simulink model "Model_Refrigeration_Constant"  (R2022a)
settings: Solver=VariableStepAuto  StartTime=0.0  StopTime=properties_8(15,2)  FixedStep=properties_8(14,2)  MaxStep=properties_8(14,2)  RelTol=1e-3  AbsTol=1e-3
InitFcn:
  | tube_D = 0.02; % [m] Refrigerant tube diameter
  | duct_W = 0.4; % [m] Air duct width
  | house_L = 4.5; % [m] House length
  | house_W = 3; % [m] House width
  | house_H = 2; % [m] House height
  | roof_pitch = 0; % [deg] Roof pitch
undefined symbols (not defined in the file or in its folder): alpha_h_ratio_NE, alpha_h_ratio_NW, alpha_h_ratio_SE, alpha_h_ratio_SW, area_furniture, area_roof, area_wall_exterior_NE, area_wall_exterior_NW, area_wall_exterior_SE, area_wall_exterior_SW, area_window, cp_furniture, cp_roof, cp_wall_exterior_NE, cp_wall_exterior_NW, cp_wall_exterior_SE, cp_wall_exterior_SW, cp_window, hc_furniture_interior, hc_roof_exterior, hc_roof_interior, hc_wall_exterior_NE, hc_wall_exterior_NW, hc_wall_exterior_SE, hc_wall_exterior_SW, hc_wall_interior_NE, hc_wall_interior_NW, hc_wall_interior_SE, hc_wall_interior_SW, hc_window_exterior, hc_window_interior, k_roof, k_wall_NE, k_wall_NW, k_wall_SE, k_wall_SW, k_window, l_roof, mass_furniture, pitch_roof, properties_8, Q_infiltration_latent, Q_infiltration_sensible, Q_latent_occupant_skin, Q_lights, Q_motor, Q_occupant, rho_roof, rho_wall_NE, rho_wall_NW, rho_wall_SE, rho_wall_SW, rho_window, SC, sigbuilder_block, T_env, T_house_init, T_init_furniture, T_set, thicnkess_roof ... (+11)
libraries: fl_lib x61, nesl_utility x15, simulink x1
(part 1 of 2)
CloseFcn:
  | try,close(h1_sscfluids_refrigeration),end
  | clear h1_sscfluids_refrigeration
  | try,close(h2_sscfluids_refrigeration),end
  | clear h2_sscfluids_refrigeration
  | try,close(h3_sscfluids_refrigeration),end
  | clear h3_sscfluids_refrigeration
  | Results
  | clear tout simlog_sscfluids_refrigeration
  | clear T_env RH_env T_house_init RH_house_init T_set
  | clear tube_D duct_W house_L house_W house_H roof_pitch
Description:
  | Refrigeration Cycle (Air Conditioning)
settings Model: Creator=The MathWorks, Inc.  LastModifiedBy=mluser
settings SolverCC: AutoScaleAbsTol=off  AlgebraicLoopSolver=TrustRegion  MaxZcPerStep=1
settings DataIOCC: ReturnWorkspaceOutputs=off
settings DebuggingCC: UnconnectedInputMsg=warning  UnconnectedOutputMsg=warning  UnconnectedLineMsg=warning  SymbolicDimsDataTypeCodeGenerationDiagnostic=none  SFMachineParentedDataDiag=warning
settings SFSimCC: CustomCodeUndefinedFunction=UseInterfaceOnly
settings RTWCC: DLArmComputeVersion=19.05
settings SimscapeCC: SimscapeLogType=all  SimscapeLogSimulationStatistics=on  SimscapeLogName=simlog_sscfluids_refrigeration  SimscapeLogDataHistory=10000

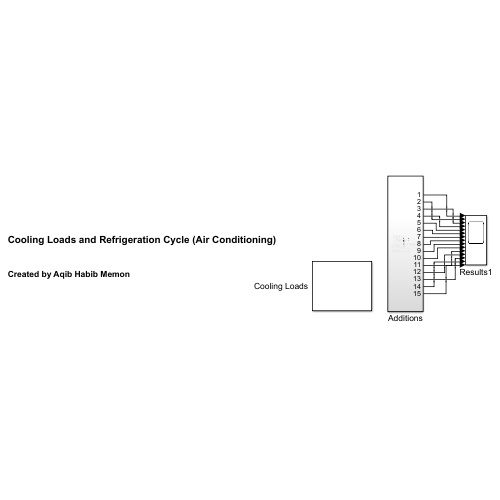
[thumbnail: Simulink's stored preview of the top-level diagram]
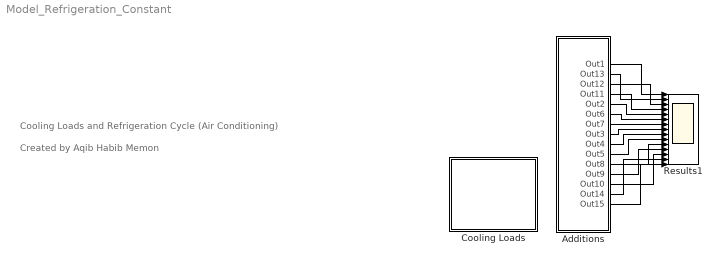
== system Model_Refrigeration_Constant ==
  note: Cooling Loads and Refrigeration Cycle (Air Conditioning)
  note: Created by Aqib Habib Memon
  Additions : Subsystem
  Cooling Loads : Subsystem
  Results1 : Scope  NumInputPorts=15
  wires:
  Additions/10(Out5) -> Results1/10
  Additions/9(Out4) -> Results1/9
  Additions/1(Out1) -> Results1/1
  Additions/2(Out13) -> Results1/2
  Additions/8(Out3) -> Results1/8
  Additions/7(Out7) -> Results1/7
  Additions/12(Out9) -> Results1/12
  Additions/5(Out2) -> Results1/5
  Additions/11(Out8) -> Results1/11
  Additions/6(Out6) -> Results1/6
  Additions/13(Out10) -> Results1/13
  Additions/3(Out12) -> Results1/3
  Additions/4(Out11) -> Results1/4
  Additions/14(Out14) -> Results1/14
  Additions/15(Out15) -> Results1/15

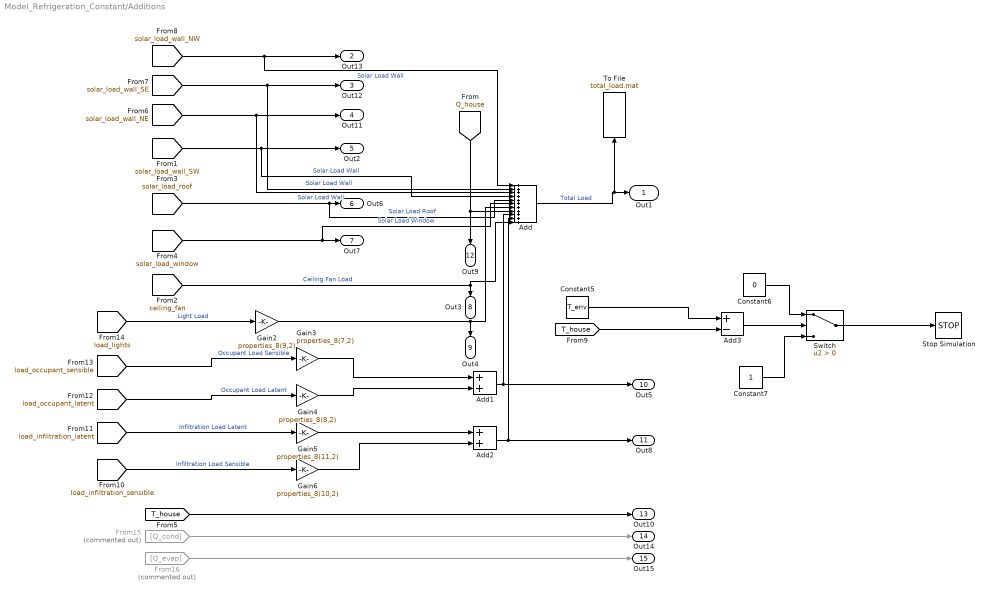
== system Model_Refrigeration_Constant/Additions ==
  Add : Sum  Inputs=+++++++++++
  Add1 : Sum
  Add2 : Sum
  Add3 : Sum  Inputs=+-
  Constant5 : Constant  Value=T_env
  Constant6 : Constant  Value=0
  Constant7 : Constant
  From15 : From  Commented=on  GotoTag=Q_cond
  From16 : From  Commented=on  GotoTag=Q_evap
  Gain2 : Gain  Gain=properties_8(9,2)
  Gain3 : Gain  Gain=properties_8(7,2)
  Gain4 : Gain  Gain=properties_8(8,2)
  Gain5 : Gain  Gain=properties_8(11,2)
  Gain6 : Gain  Gain=properties_8(10,2)
  Stop Simulation : Stop
  Switch : Switch  Criteria=u2 > Threshold  SaturateOnIntegerOverflow=off  InputSameDT=off
  To File : ToFile  Filename=total_load.mat  MatrixName=total_load
  Out1 : Outport
  Out13 : Outport  Port=2
  Out12 : Outport  Port=3
  Out11 : Outport  Port=4
  Out2 : Outport  Port=5
  Out6 : Outport  Port=6
  Out7 : Outport  Port=7
  Out3 : Outport  Port=8
  Out4 : Outport  Port=9
  Out5 : Outport  Port=10
  Out8 : Outport  Port=11
  Out9 : Outport  Port=12
  Out10 : Outport  Port=13
  Out14 : Outport  Port=14
  Out15 : Outport  Port=15
  wires:
  [load_lights] -> Gain2/1  "Light Load"
  [ceiling_fan] -> Add/11, Out3/1  "Ceiling Fan Load"
  Add/1 -> Out1/1, To File/1  "Total Load"
  [load_occupant_sensible] -> Gain3/1  "Occupant Load Sensible"
  [load_occupant_latent] -> Gain4/1  "Occupant Load Latent"
  [load_infiltration_sensible] -> Gain6/1  "Infiltration Load Sensible"
  [Q_house] -> Add/8, Out9/1
  [solar_load_wall_SW] -> Add/4, Out2/1  "Solar Load Wall"
  [solar_load_roof] -> Add/5, Out6/1  "Solar Load Roof"
  [solar_load_window] -> Add/6, Out7/1  "Solar Load Window"
  [T_house] -> Out10/1
  [solar_load_wall_NE] -> Add/3, Out11/1  "Solar Load Wall"
  [solar_load_wall_SE] -> Add/2, Out12/1  "Solar Load Wall"
  [solar_load_wall_NW] -> Add/1, Out13/1  "Solar Load Wall"
  [load_infiltration_latent] -> Gain5/1  "Infiltration Load Latent"
  Add1/1 -> Out5/1, Add/9
  Add2/1 -> Add/10, Out8/1
  Gain2/1 -> Add/7, Out4/1
  Gain3/1 -> Add1/1
  Gain4/1 -> Add1/2
  Gain5/1 -> Add2/1
  Gain6/1 -> Add2/2
  Constant5/1 -> Add3/1
  [T_house] -> Add3/2
  Add3/1 -> Switch/2
  Constant6/1 -> Switch/1
  Constant7/1 -> Switch/3
  Switch/1 -> Stop Simulation/1
  From16/1 -> Out15/1
  From15/1 -> Out14/1

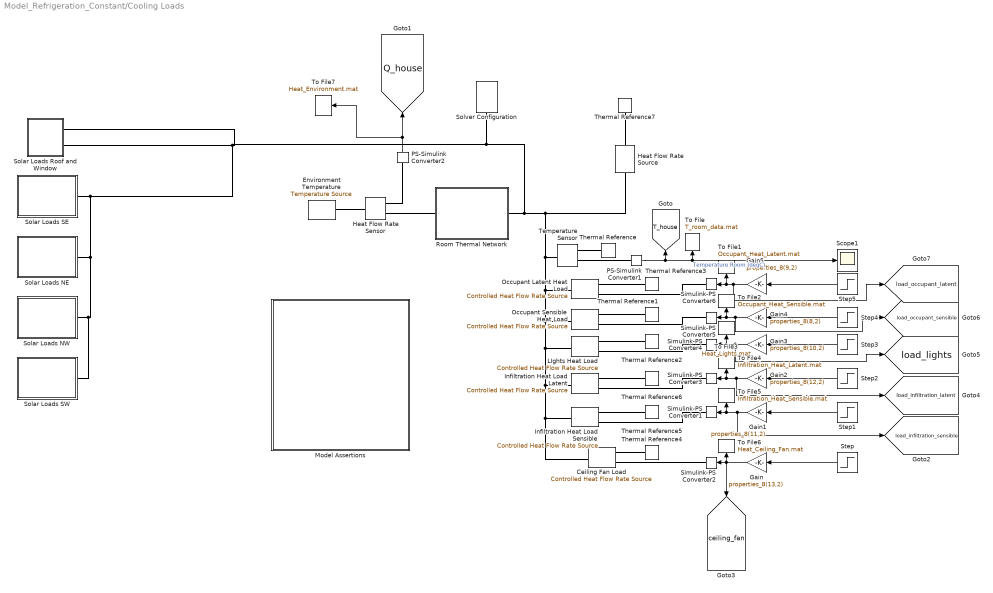
== system Model_Refrigeration_Constant/Cooling Loads ==
  Ceiling Fan Load : fl_lib/Thermal/Thermal Sources/Controlled Heat Flow Rate Source
      settings: SourceProductBaseCode=PW,SS,VE
  Environment Temperature : fl_lib/Thermal/Thermal Sources/Temperature Source  temperature=T_env degC
      settings: SourceProductBaseCode=PW,SS,VE
  Gain : Gain  Gain=properties_8(13,2)
  Gain1 : Gain  Gain=properties_8(11,2)
  Gain2 : Gain  Gain=properties_8(12,2)
  Gain3 : Gain  Gain=properties_8(10,2)
  Gain4 : Gain  Gain=properties_8(8,2)
  Gain5 : Gain  Gain=properties_8(9,2)
  Heat Flow Rate Sensor : fl_lib/Thermal/Thermal Sensors/Heat Flow Rate Sensor
      settings: SourceProductBaseCode=PW,SS,VE
  Heat Flow Rate Source : fl_lib/Thermal/Thermal Sources/Heat Flow Rate Source  heat_flow=5250 W
      settings: SourceProductBaseCode=PW,SS,VE  InternalSimscapePortConfiguration="{\"Bottom\":[],\"Left\":[{\"id\":\"B\",\"label\":\"B\",\"type\":\"foundation.thermal.thermal\"}],\"Right\":[{\"id\":\"A\",\"label\":\"A\",\"type\":\"foundation.thermal.thermal\"}],\"Top\":[]}"
  Infiltration Heat Load Latent : fl_lib/Thermal/Thermal Sources/Controlled Heat Flow Rate Source
      settings: SourceProductBaseCode=PW,SS,VE
  Infiltration Heat Load Sensible : fl_lib/Thermal/Thermal Sources/Controlled Heat Flow Rate Source
      settings: SourceProductBaseCode=PW,SS,VE
  LIghts Heat Load : fl_lib/Thermal/Thermal Sources/Controlled Heat Flow Rate Source
      settings: SourceProductBaseCode=PW,SS,VE
  Model Assertions : Subsystem
  Occupant Latent Heat Load : fl_lib/Thermal/Thermal Sources/Controlled Heat Flow Rate Source
      settings: SourceProductBaseCode=PW,SS,VE
  Occupant Sensible Heat Load : fl_lib/Thermal/Thermal Sources/Controlled Heat Flow Rate Source
      settings: SourceProductBaseCode=PW,SS,VE
  PS-Simulink Converter1 : nesl_utility/PS-Simulink Converter  PhysicalDomain=network_engine_domain  SubClassName=ps_output  LeftPortType=input  RightPortType=output  PseudoPeriodic=off  Frequencies=[]  VectorFormat=inherit  Unit=degC  AffineConversion=on
      settings: SourceProductBaseCode=SS,PW,VE
  PS-Simulink Converter2 : nesl_utility/PS-Simulink Converter  PhysicalDomain=network_engine_domain  SubClassName=ps_output  LeftPortType=input  RightPortType=output  PseudoPeriodic=off  Frequencies=[]  VectorFormat=inherit  Unit=W  AffineConversion=off
      settings: SourceProductBaseCode=SS,PW,VE
  Room Thermal Network : Subsystem  Tag=PublishSubsystem  mask(House Thermal Network){area_roof=l_roof * w_roof / (2*cosd(pitch_roof)), thickness_roof=thicnkess_roof, rho_roof=rho_roof, cp_roof=cp_roof, k_roof=k_roof, hc_roof_interior=hc_roof_interior, hc_roof_exterior=hc_roof_exterior, T_init_roof=T_house_init, area_wall_SE=area_wall_exterior_SE, thickness_wall_SE=thicnkess_wall_exterior_SE, rho_wall_SE=rho_wall_SE, cp_wall_SE=cp_wall_exterior_SE, k_wall_SE=k_wall_SE, hc_wall_interior_SE=hc_wall_interior_SE, hc_wall_exterior_SE=hc_wall_exterior_SE, T_init_wall_SE=T_house_init, area_wall_NE=area_wall_exterior_NE, thickness_wall_copy_NE=thicnkess_wall_exterior_NE, rho_wall_NE=rho_wall_NE, cp_wall_NE=cp_wall_exterior_NE, k_wall_NE=k_wall_NE, hc_wall_interior_NE=hc_wall_interior_NE, hc_wall_exterior_NE=hc_wall_exterior_NE, T_init_wall_NE=T_house_init, area_wall_SW=area_wall_exterior_SW, thickness_wall_SW=thicnkess_wall_exterior_SW, rho_wal_SW=rho_wall_SW, cp_wall_SW=cp_wall_exterior_SW, k_wall_SW=k_wall_SW, hc_wall_SW=hc_wall_interior_SW, hc_wall_exterior_SW=hc_wall_exterior_SW, T_init_wall_SW=T_house_init, area_wall_NW=area_wall_exterior_NW, thickness_wall_NW=thicnkess_wall_exterior_NW, rho_wall_NW=rho_wall_NW, cp_wall_NW=cp_wall_exterior_NW, k_wall_NW=k_wall_NW, hc_wall_interior_NW=hc_wall_interior_NW, hc_wall_exterior_NW=hc_wall_exterior_NW, T_init_wall_NW=T_house_init, area_window=area_window, thickness_window=thicnkess_window, rho_window=rho_window, cp_window=cp_window, k_window=k_window, hc_window_interior=hc_window_interior, hc_window_exterior=hc_window_exterior, T_init_window=T_house_init, area_furniture=area_furniture, M_furniture=mass_furniture, cp_furniture=cp_furniture, hc_furniture_interior=hc_furniture_interior, T_init_furniture=T_init_furniture}
      mask prompts: area_roof "Total area (m^2)"; thickness_roof "Average thickness (m)"; rho_roof "Average density (kg/m^3)"; cp_roof "Average specific heat (J/kg/K)"; k_roof "Average conductivity (W/m/K)"; hc_roof_interior "Interior heat transfer coefficient (W/m^2/K)"; hc_roof_exterior "Exterior heat transfer coefficient (W/m^2/K)"; T_init_roof "Initial temperature (degC)"; area_wall_SE "Total area (m^2)"; thickness_wall_SE "Average thickness (m)"; rho_wall_SE "Average density (kg/m^3)"; cp_wall_SE "Average specific heat (J/kg/K)"; k_wall_SE "Average conductivity (W/m/K)"; hc_wall_interior_SE "Interior heat transfer coefficient (W/m^2/K)"; hc_wall_exterior_SE "Exterior heat transfer coefficient (W/m^2/K)"; T_init_wall_SE "Initial temperature (degC)"; area_wall_NE "Total area (m^2)"; thickness_wall_copy_NE "Average thickness (m)"; rho_wall_NE "Average density (kg/m^3)"; cp_wall_NE "Average specific heat (J/kg/K)"; k_wall_NE "Average conductivity (W/m/K)"; hc_wall_interior_NE "Interior heat transfer coefficient (W/m^2/K)"; hc_wall_exterior_NE "Exterior heat transfer coefficient (W/m^2/K)"; T_init_wall_NE "Initial temperature (degC)"; area_wall_SW "Total area (m^2)"; thickness_wall_SW "Average thickness (m)"; rho_wal_SW "Average density (kg/m^3)"; cp_wall_SW "Average specific heat (J/kg/K)"; k_wall_SW "Average conductivity (W/m/K)"; hc_wall_SW "Interior heat transfer coefficient (W/m^2/K)"; hc_wall_exterior_SW "Exterior heat transfer coefficient (W/m^2/K)"; T_init_wall_SW "Initial temperature (degC)"; area_wall_NW "Total area (m^2)"; thickness_wall_NW "Average thickness (m)"; rho_wall_NW "Average density (kg/m^3)"; cp_wall_NW "Average specific heat (J/kg/K)"; k_wall_NW "Average conductivity (W/m/K)"; hc_wall_interior_NW "Interior heat transfer coefficient (W/m^2/K)"; hc_wall_exterior_NW "Exterior heat transfer coefficient (W/m^2/K)"; T_init_wall_NW "Initial temperature (degC)"; area_window "Total area (m^2)"; thickness_window "Average thickness (m)"; rho_window "Average density (kg/m^3)"; cp_window "Average specific heat (J/kg/K)"; k_window "Average conductivity (W/m/K)"; hc_window_interior "Interior heat transfer coefficient (W/m^2/K)"; hc_window_exterior "Exterior heat transfer coefficient (W/m^2/K)"; T_init_window "Initial temperature (degC)"; area_furniture "Total surface area (m^2)"; M_furniture "Total mass (kg)"; cp_furniture "Average specific heat (J/kg/K)"; hc_furniture_interior "Interior heat transfer coefficient (W/m^2/K)"; T_init_furniture "Initial temperature (degC)"
      mask help: This subsystem models heat transfer between the air in the interior of the house and the external environment.
      mask DialogControl TabRoof Prompt: Roof
      mask DialogControl TabWallSE Prompt: South East Walls
      mask DialogControl TabWallNE Prompt: North East Walls
      mask DialogControl TabWallSW Prompt: South West Walls
      mask DialogControl TabWallNW Prompt: North West Walls
      mask DialogControl TabWindow Prompt: Windows
      mask DialogControl TabFurniture Prompt: Furniture
  Scope1 : Scope
  Simulink-PS Converter{1..6} (6 alike) : nesl_utility/Simulink-PS Converter  PhysicalDomain=network_engine_domain  SubClassName=ps_input  LeftPortType=input  RightPortType=output  PseudoPeriodic=off  Frequencies=[]  NoiseDistribution=none  NoiseParameters=[]  Unit=1  AffineConversion=off  FilteringAndDerivatives=provide  SimscapeFilterOrder=1  InputFilterTimeConstant=0.001  UdotUserProvided=0
      settings: SourceProductBaseCode=SS,PW,VE
  Solar Loads NE : Subsystem
  Solar Loads NW : Subsystem
  Solar Loads Roof and Window : Subsystem
  Solar Loads SE : Subsystem
  Solar Loads SW : Subsystem
  Solver Configuration : nesl_utility/Solver Configuration  PhysicalDomain=network_engine_domain  SubClassName=solver  LeftPortType=input  RightPortType=generic  Tones=[]  Harmonics=[]  SimulateNoise=off  Profile=off  UseLocalSampling=off  EnableSwitchedLinearOptims=on  FrequencyDomain=off  UseCCode=off  RelTol=0.001  AbsTol=0.001  MinStep=1e-09  ToWorkspace=off  RevertToSquareIcSolve=off  NumHomotopyIterations=100  PhasorMode=off  PhasorModeNumHarmonics=1  IndexReductionMethod=DerivativeReplacement  DoDC=off  ResidualTolerance=1e-09  UseLocalSolver=off  LocalSolverChoice=NE_BACKWARD_EULER_ADVANCER  LocalSolverSampleTime=0.001  DoFixedCost=off  MaxNonlinIter=3  MaxModeIter=2  ComputeImpulses=off  ImpulseIterations=2  LinearAlgebra=auto  LinearAlgebraNumThread=0  EquationFormulation=NE_TIME_EF  DelaysMemoryBudget=1024  AutomaticFiltering=on  FilteringTimeConstant=0.001  PartitionStorageMethod=AS_NEEDED  PartitionMemoryBudget=1024  PartitionMethod=ROBUST
      settings: SourceProductBaseCode=SS,PW,VE
  Step : Step  Time=0  After=Q_motor  SampleTime=0
  Step1 : Step  Time=0  After=Q_infiltration_sensible  SampleTime=0
  Step2 : Step  Time=0  After=Q_infiltration_latent  SampleTime=0
  Step3 : Step  Time=0  After=Q_lights  SampleTime=0
  Step4 : Step  Time=0  After=Q_occupant  SampleTime=0
  Step5 : Step  Time=0  After=Q_latent_occupant_skin  SampleTime=0
  Temperature Sensor : fl_lib/Thermal/Thermal Sensors/Temperature Sensor
      settings: SourceProductBaseCode=PW,SS,VE
  Thermal Reference{,1..7} (8 alike) : fl_lib/Thermal/Thermal Elements/Thermal Reference
      settings: SourceProductBaseCode=PW,SS,VE
  To File : ToFile  Filename=T_room_data.mat  MatrixName=T_room_data
  To File1 : ToFile  Filename=Occupant_Heat_Latent.mat  MatrixName=Occupant_Heat_Latent
  To File2 : ToFile  Filename=Occupant_Heat_Sensible.mat  MatrixName=Occupant_Heat_Sensible
  To File3 : ToFile  Filename=Heat_Lights.mat  MatrixName=Heat_Lights
  To File4 : ToFile  Filename=Infiltration_Heat_Latent.mat  MatrixName=Infiltration_Heat_Latent
  To File5 : ToFile  Filename=Infiltration_Heat_Sensible.mat  MatrixName=Infiltration_Heat_Sensible
  To File6 : ToFile  Filename=Heat_Ceiling_Fan.mat  MatrixName=Heat_Ceiling_Fan
  To File7 : ToFile  Filename=Heat_Environment.mat  MatrixName=Heat_Environment
  tag scope: Q_house=global, T_house=global, ceiling_fan=global, load_infiltration_latent=global, load_infiltration_sensible=global, load_lights=global, load_occupant_latent=global, load_occupant_sensible=global
  wires:
  PS-Simulink Converter1/1 -> Scope1/1, To File/1, [T_house]  "Temperature Room (degC)"
  PS-Simulink Converter2/1 -> To File7/1, [Q_house]
  Gain/1 -> To File6/1, [ceiling_fan], Simulink-PS Converter2/1
  Step/1 -> Gain/1
  Step1/1 -> Gain1/1
  Step2/1 -> Gain2/1
  Step3/1 -> Gain3/1
  Step4/1 -> Gain4/1
  Step5/1 -> Gain5/1
  Gain5/1 -> Simulink-PS Converter6/1, To File1/1, [load_occupant_latent]
  Gain4/1 -> [load_occupant_sensible], To File2/1, Simulink-PS Converter5/1
  Gain3/1 -> [load_lights], To File3/1, Simulink-PS Converter4/1
  Gain2/1 -> [load_infiltration_latent], To File4/1, Simulink-PS Converter3/1
  Gain1/1 -> [load_infiltration_sensible], To File5/1, Simulink-PS Converter1/1
  connections:
  Temperature Sensor/RConn2 -- PS-Simulink Converter1/LConn1
  Temperature Sensor/RConn1 -- Thermal Reference/LConn1
  Solar Loads SW/RConn1 -- Solar Loads NW/RConn1 -- Solar Loads NE/RConn1 -- Solar Loads Roof and Window/RConn1 -- Solver Configuration/RConn1 -- Heat Flow Rate Source/RConn1 -- Ceiling Fan Load/LConn1 -- Infiltration Heat Load Sensible/LConn1 -- Infiltration Heat Load Latent/LConn1 -- LIghts Heat Load/LConn1 -- Occupant Sensible Heat Load/LConn1 -- Occupant Latent Heat Load/LConn1 -- Temperature Sensor/LConn1 -- Room Thermal Network/RConn1 -- Solar Loads Roof and Window/RConn2 -- Solar Loads SE/RConn1
  Thermal Reference4/LConn1 -- Ceiling Fan Load/RConn2
  Simulink-PS Converter2/RConn1 -- Ceiling Fan Load/RConn1
  Heat Flow Rate Sensor/LConn1 -- Environment Temperature/LConn1
  PS-Simulink Converter2/LConn1 -- Heat Flow Rate Sensor/RConn1
  Occupant Latent Heat Load/RConn2 -- Thermal Reference3/LConn1
  Occupant Sensible Heat Load/RConn2 -- Thermal Reference1/LConn1
  LIghts Heat Load/RConn2 -- Thermal Reference2/LConn1
  Infiltration Heat Load Sensible/RConn2 -- Thermal Reference5/LConn1
  Thermal Reference6/LConn1 -- Infiltration Heat Load Latent/RConn2
  Simulink-PS Converter6/RConn1 -- Occupant Latent Heat Load/RConn1
  Simulink-PS Converter5/RConn1 -- Occupant Sensible Heat Load/RConn1
  Simulink-PS Converter4/RConn1 -- LIghts Heat Load/RConn1
  Simulink-PS Converter3/RConn1 -- Infiltration Heat Load Latent/RConn1
  Simulink-PS Converter1/RConn1 -- Infiltration Heat Load Sensible/RConn1
  Heat Flow Rate Sensor/RConn2 -- Room Thermal Network/LConn1
  Thermal Reference7/LConn1 -- Heat Flow Rate Source/LConn1

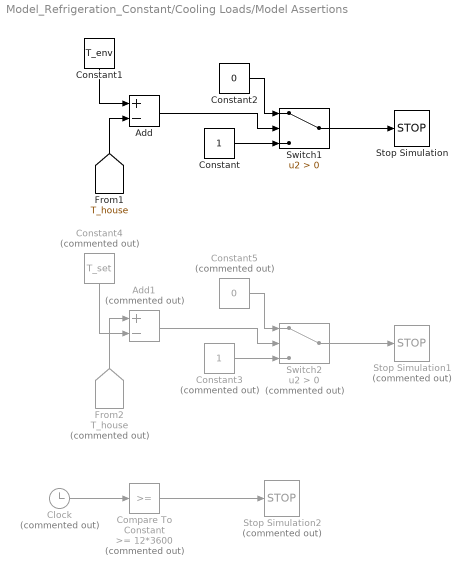
== system Model_Refrigeration_Constant/Cooling Loads/Model Assertions ==
  Add : Sum  Inputs=+-
  Add1 : Sum  Commented=on  Inputs=+-
  Clock : Clock  Commented=on
  Compare To Constant : simulink/Logic and Bit Operations/Compare To Constant  Commented=on  relop=>=  const=12*3600  OutDataTypeStr=boolean
  Constant : Constant
  Constant1 : Constant  Value=T_env
  Constant2 : Constant  Value=0
  Constant3 : Constant  Commented=on
  Constant4 : Constant  Commented=on  Value=T_set
  Constant5 : Constant  Commented=on  Value=0
  From2 : From  Commented=on  GotoTag=T_house  TagVisibility=global
  Stop Simulation : Stop
  Stop Simulation1 : Stop  Commented=on
  Stop Simulation2 : Stop  Commented=on
  Switch1 : Switch  Criteria=u2 > Threshold  SaturateOnIntegerOverflow=off  InputSameDT=off
  Switch2 : Switch  Commented=on  Criteria=u2 > Threshold  SaturateOnIntegerOverflow=off  InputSameDT=off
  wires:
  Constant/1 -> Switch1/3
  Constant3/1 -> Switch2/3
  [T_house] -> Add/2
  Constant4/1 -> Add1/2
  Constant2/1 -> Switch1/1
  Switch1/1 -> Stop Simulation/1
  Add1/1 -> Switch2/2
  Constant5/1 -> Switch2/1
  Add/1 -> Switch1/2
  Switch2/1 -> Stop Simulation1/1
  Constant1/1 -> Add/1
  From2/1 -> Add1/1
  Compare To Constant/1 -> Stop Simulation2/1
  Clock/1 -> Compare To Constant/1

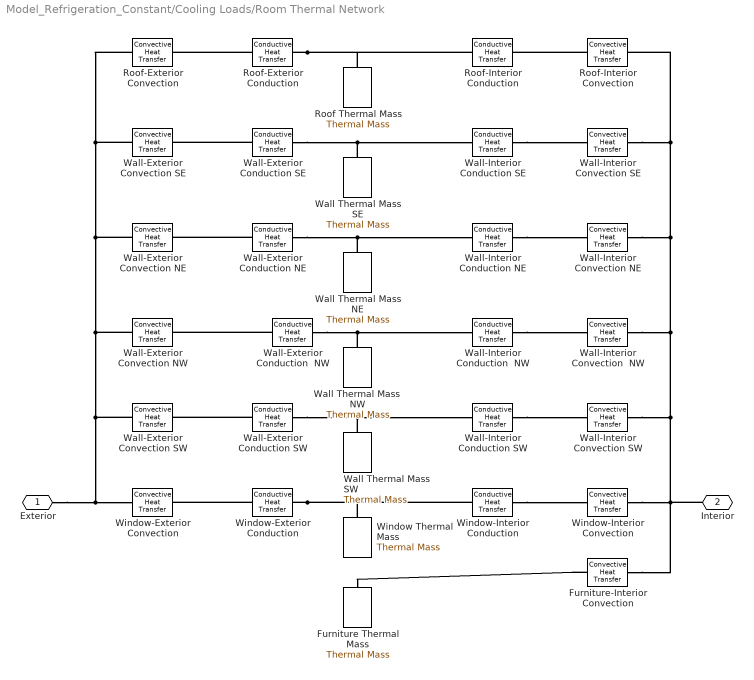
== system Model_Refrigeration_Constant/Cooling Loads/Room Thermal Network ==
  Furniture Thermal Mass : fl_lib/Thermal/Thermal Elements/Thermal Mass  mass=M_furniture kg  sp_heat=cp_furniture J/(K*kg)  T_specify=on  T_priority=High  T=T_init_furniture degC  T_nominal_specify=off  T_nominal_unit=K  T_nominal_value=1  Q_specify=off  Q_priority=None  Q=0 W  Q_nominal_specify=off  Q_nominal_unit=W  Q_nominal_value=1
      settings: SourceProductBaseCode=PW,SS,VE
  Furniture-Interior Convection : fl_lib/Thermal/Thermal Elements/Convective Heat Transfer  area=area_furniture m^2  heat_tr_coeff=hc_furniture_interior W/(K*m^2)  T_specify=off  T_priority=None  T=0 K  T_nominal_specify=off  T_nominal_unit=K  T_nominal_value=1  Q_specify=off  Q_priority=None  Q=0 W  Q_nominal_specify=off  Q_nominal_unit=W  Q_nominal_value=1
      settings: SourceProductBaseCode=PW,SS,VE
  Roof Thermal Mass : fl_lib/Thermal/Thermal Elements/Thermal Mass  mass=rho_roof * area_roof * thickness_roof kg  sp_heat=cp_roof J/(K*kg)  T_specify=on  T_priority=High  T=T_init_roof degC  T_nominal_specify=off  T_nominal_unit=K  T_nominal_value=1  Q_specify=off  Q_priority=None  Q=0 W  Q_nominal_specify=off  Q_nominal_unit=W  Q_nominal_value=1
      settings: SourceProductBaseCode=PW,SS,VE
  Roof-Exterior Conduction : fl_lib/Thermal/Thermal Elements/Conductive Heat Transfer  area=area_roof m^2  thickness=thickness_roof / 2 m  th_cond=k_roof W/(K*m)  T_specify=off  T_priority=None  T=0 K  T_nominal_specify=off  T_nominal_unit=K  T_nominal_value=1  Q_specify=off  Q_priority=None  Q=0 W  Q_nominal_specify=off  Q_nominal_unit=W  Q_nominal_value=1
      settings: SourceProductBaseCode=PW,SS,VE
  Roof-Exterior Convection : fl_lib/Thermal/Thermal Elements/Convective Heat Transfer  area=area_roof m^2  heat_tr_coeff=hc_roof_exterior W/(K*m^2)  T_specify=off  T_priority=None  T=0 K  T_nominal_specify=off  T_nominal_unit=K  T_nominal_value=1  Q_specify=off  Q_priority=None  Q=0 W  Q_nominal_specify=off  Q_nominal_unit=W  Q_nominal_value=1
      settings: SourceProductBaseCode=PW,SS,VE
  Roof-Interior Conduction : fl_lib/Thermal/Thermal Elements/Conductive Heat Transfer  area=area_roof m^2  thickness=thickness_roof / 2 m  th_cond=k_roof W/(K*m)  T_specify=off  T_priority=None  T=0 K  T_nominal_specify=off  T_nominal_unit=K  T_nominal_value=1  Q_specify=off  Q_priority=None  Q=0 W  Q_nominal_specify=off  Q_nominal_unit=W  Q_nominal_value=1
      settings: SourceProductBaseCode=PW,SS,VE
  Roof-Interior Convection : fl_lib/Thermal/Thermal Elements/Convective Heat Transfer  area=area_roof m^2  heat_tr_coeff=hc_roof_interior W/(K*m^2)  T_specify=off  T_priority=None  T=0 K  T_nominal_specify=off  T_nominal_unit=K  T_nominal_value=1  Q_specify=off  Q_priority=None  Q=0 W  Q_nominal_specify=off  Q_nominal_unit=W  Q_nominal_value=1
      settings: SourceProductBaseCode=PW,SS,VE
  Wall Thermal Mass  NW : fl_lib/Thermal/Thermal Elements/Thermal Mass  mass=mass_wall_exterior_NW kg  sp_heat=cp_wall_NW J/(K*kg)  T_specify=on  T_priority=High  T=T_init_wall_NW degC  T_nominal_specify=off  T_nominal_unit=K  T_nominal_value=1  Q_specify=off  Q_priority=None  Q=0 W  Q_nominal_specify=off  Q_nominal_unit=W  Q_nominal_value=1
      settings: SourceProductBaseCode=PW,SS,VE
  Wall Thermal Mass NE : fl_lib/Thermal/Thermal Elements/Thermal Mass  mass=mass_wall_exterior_NE kg  sp_heat=cp_wall_NE J/(K*kg)  T_specify=on  T_priority=High  T=T_init_wall_NE degC  T_nominal_specify=off  T_nominal_unit=K  T_nominal_value=1  Q_specify=off  Q_priority=None  Q=0 W  Q_nominal_specify=off  Q_nominal_unit=W  Q_nominal_value=1
      settings: SourceProductBaseCode=PW,SS,VE
  Wall Thermal Mass SE : fl_lib/Thermal/Thermal Elements/Thermal Mass  mass=mass_wall_exterior_SE kg  sp_heat=cp_wall_SE J/(K*kg)  T_specify=on  T_priority=High  T=T_init_wall_SE degC  T_nominal_specify=off  T_nominal_unit=K  T_nominal_value=1  Q_specify=off  Q_priority=None  Q=0 W  Q_nominal_specify=off  Q_nominal_unit=W  Q_nominal_value=1
      settings: SourceProductBaseCode=PW,SS,VE
  Wall Thermal Mass SW : fl_lib/Thermal/Thermal Elements/Thermal Mass  mass=mass_wall_exterior_SW kg  sp_heat=cp_wall_SW J/(K*kg)  T_specify=on  T_priority=High  T=T_init_wall_SW degC  T_nominal_specify=off  T_nominal_unit=K  T_nominal_value=1  Q_specify=off  Q_priority=None  Q=0 W  Q_nominal_specify=off  Q_nominal_unit=W  Q_nominal_value=1
      settings: SourceProductBaseCode=PW,SS,VE
  Wall-Exterior Conduction  NW : fl_lib/Thermal/Thermal Elements/Conductive Heat Transfer  area=area_wall_NW m^2  thickness=thicnkess_wall_exterior_NW / 2 m  th_cond=k_wall_NW W/(K*m)  T_specify=off  T_priority=None  T=0 K  T_nominal_specify=off  T_nominal_unit=K  T_nominal_value=1  Q_specify=off  Q_priority=None  Q=0 W  Q_nominal_specify=off  Q_nominal_unit=W  Q_nominal_value=1
      settings: SourceProductBaseCode=PW,SS,VE
  Wall-Exterior Conduction NE : fl_lib/Thermal/Thermal Elements/Conductive Heat Transfer  area=area_wall_NE m^2  thickness=thicnkess_wall_exterior_NE / 2 m  th_cond=k_wall_NE W/(K*m)  T_specify=off  T_priority=None  T=0 K  T_nominal_specify=off  T_nominal_unit=K  T_nominal_value=1  Q_specify=off  Q_priority=None  Q=0 W  Q_nominal_specify=off  Q_nominal_unit=W  Q_nominal_value=1
      settings: SourceProductBaseCode=PW,SS,VE
  Wall-Exterior Conduction SE : fl_lib/Thermal/Thermal Elements/Conductive Heat Transfer  area=area_wall_SE m^2  thickness=thicnkess_wall_exterior_SE / 2 m  th_cond=k_wall_SE W/(K*m)  T_specify=off  T_priority=None  T=0 K  T_nominal_specify=off  T_nominal_unit=K  T_nominal_value=1  Q_specify=off  Q_priority=None  Q=0 W  Q_nominal_specify=off  Q_nominal_unit=W  Q_nominal_value=1
      settings: SourceProductBaseCode=PW,SS,VE
  Wall-Exterior Conduction SW : fl_lib/Thermal/Thermal Elements/Conductive Heat Transfer  area=area_wall_SW m^2  thickness=thicnkess_wall_exterior_SW / 2 m  th_cond=k_wall_SW W/(K*m)  T_specify=off  T_priority=None  T=0 K  T_nominal_specify=off  T_nominal_unit=K  T_nominal_value=1  Q_specify=off  Q_priority=None  Q=0 W  Q_nominal_specify=off  Q_nominal_unit=W  Q_nominal_value=1
      settings: SourceProductBaseCode=PW,SS,VE
  Wall-Exterior Convection NE : fl_lib/Thermal/Thermal Elements/Convective Heat Transfer  area=area_wall_NE m^2  heat_tr_coeff=hc_wall_exterior_NE W/(K*m^2)  T_specify=off  T_priority=None  T=0 K  T_nominal_specify=off  T_nominal_unit=K  T_nominal_value=1  Q_specify=off  Q_priority=None  Q=0 W  Q_nominal_specify=off  Q_nominal_unit=W  Q_nominal_value=1
      settings: SourceProductBaseCode=PW,SS,VE
  Wall-Exterior Convection NW : fl_lib/Thermal/Thermal Elements/Convective Heat Transfer  area=area_wall_NW m^2  heat_tr_coeff=hc_wall_exterior_NW W/(K*m^2)  T_specify=off  T_priority=None  T=0 K  T_nominal_specify=off  T_nominal_unit=K  T_nominal_value=1  Q_specify=off  Q_priority=None  Q=0 W  Q_nominal_specify=off  Q_nominal_unit=W  Q_nominal_value=1
      settings: SourceProductBaseCode=PW,SS,VE
  Wall-Exterior Convection SE : fl_lib/Thermal/Thermal Elements/Convective Heat Transfer  area=area_wall_SE m^2  heat_tr_coeff=hc_wall_exterior_SE W/(K*m^2)  T_specify=off  T_priority=None  T=0 K  T_nominal_specify=off  T_nominal_unit=K  T_nominal_value=1  Q_specify=off  Q_priority=None  Q=0 W  Q_nominal_specify=off  Q_nominal_unit=W  Q_nominal_value=1
      settings: SourceProductBaseCode=PW,SS,VE
  Wall-Exterior Convection SW : fl_lib/Thermal/Thermal Elements/Convective Heat Transfer  area=area_wall_SW m^2  heat_tr_coeff=hc_wall_exterior_SW W/(K*m^2)  T_specify=off  T_priority=None  T=0 K  T_nominal_specify=off  T_nominal_unit=K  T_nominal_value=1  Q_specify=off  Q_priority=None  Q=0 W  Q_nominal_specify=off  Q_nominal_unit=W  Q_nominal_value=1
      settings: SourceProductBaseCode=PW,SS,VE
  Wall-Interior Conduction  NW : fl_lib/Thermal/Thermal Elements/Conductive Heat Transfer  area=area_wall_NW m^2  thickness=thicnkess_wall_exterior_NW/ 2 m  th_cond=k_wall_NW W/(K*m)  T_specify=off  T_priority=None  T=0 K  T_nominal_specify=off  T_nominal_unit=K  T_nominal_value=1  Q_specify=off  Q_priority=None  Q=0 W  Q_nominal_specify=off  Q_nominal_unit=W  Q_nominal_value=1
      settings: SourceProductBaseCode=PW,SS,VE
  Wall-Interior Conduction NE : fl_lib/Thermal/Thermal Elements/Conductive Heat Transfer  area=area_wall_NE m^2  thickness=thicnkess_wall_exterior_NE/ 2 m  th_cond=k_wall_NE W/(K*m)  T_specify=off  T_priority=None  T=0 K  T_nominal_specify=off  T_nominal_unit=K  T_nominal_value=1  Q_specify=off  Q_priority=None  Q=0 W  Q_nominal_specify=off  Q_nominal_unit=W  Q_nominal_value=1
      settings: SourceProductBaseCode=PW,SS,VE
  Wall-Interior Conduction SE : fl_lib/Thermal/Thermal Elements/Conductive Heat Transfer  area=area_wall_SE m^2  thickness=thicnkess_wall_exterior_SE/ 2 m  th_cond=k_wall_SE W/(K*m)  T_specify=off  T_priority=None  T=0 K  T_nominal_specify=off  T_nominal_unit=K  T_nominal_value=1  Q_specify=off  Q_priority=None  Q=0 W  Q_nominal_specify=off  Q_nominal_unit=W  Q_nominal_value=1
      settings: SourceProductBaseCode=PW,SS,VE
  Wall-Interior Conduction SW : fl_lib/Thermal/Thermal Elements/Conductive Heat Transfer  area=area_wall_SW m^2  thickness=thicnkess_wall_exterior_SW/ 2 m  th_cond=k_wall_SW W/(K*m)  T_specify=off  T_priority=None  T=0 K  T_nominal_specify=off  T_nominal_unit=K  T_nominal_value=1  Q_specify=off  Q_priority=None  Q=0 W  Q_nominal_specify=off  Q_nominal_unit=W  Q_nominal_value=1
      settings: SourceProductBaseCode=PW,SS,VE
  Wall-Interior Convection  NW : fl_lib/Thermal/Thermal Elements/Convective Heat Transfer  area=area_wall_NW m^2  heat_tr_coeff=hc_wall_interior_NW W/(K*m^2)  T_specify=off  T_priority=None  T=0 K  T_nominal_specify=off  T_nominal_unit=K  T_nominal_value=1  Q_specify=off  Q_priority=None  Q=0 W  Q_nominal_specify=off  Q_nominal_unit=W  Q_nominal_value=1
      settings: SourceProductBaseCode=PW,SS,VE
  Wall-Interior Convection NE : fl_lib/Thermal/Thermal Elements/Convective Heat Transfer  area=area_wall_NE m^2  heat_tr_coeff=hc_wall_interior_NE W/(K*m^2)  T_specify=off  T_priority=None  T=0 K  T_nominal_specify=off  T_nominal_unit=K  T_nominal_value=1  Q_specify=off  Q_priority=None  Q=0 W  Q_nominal_specify=off  Q_nominal_unit=W  Q_nominal_value=1
      settings: SourceProductBaseCode=PW,SS,VE
  Wall-Interior Convection SE : fl_lib/Thermal/Thermal Elements/Convective Heat Transfer  area=area_wall_SE m^2  heat_tr_coeff=hc_wall_interior_SE W/(K*m^2)  T_specify=off  T_priority=None  T=0 K  T_nominal_specify=off  T_nominal_unit=K  T_nominal_value=1  Q_specify=off  Q_priority=None  Q=0 W  Q_nominal_specify=off  Q_nominal_unit=W  Q_nominal_value=1
      settings: SourceProductBaseCode=PW,SS,VE
  Wall-Interior Convection SW : fl_lib/Thermal/Thermal Elements/Convective Heat Transfer  area=area_wall_SW m^2  heat_tr_coeff=hc_wall_interior_SW W/(K*m^2)  T_specify=off  T_priority=None  T=0 K  T_nominal_specify=off  T_nominal_unit=K  T_nominal_value=1  Q_specify=off  Q_priority=None  Q=0 W  Q_nominal_specify=off  Q_nominal_unit=W  Q_nominal_value=1
      settings: SourceProductBaseCode=PW,SS,VE
  Window Thermal Mass : fl_lib/Thermal/Thermal Elements/Thermal Mass  mass=rho_window * area_window * thickness_window kg  sp_heat=cp_window J/(K*kg)  T_specify=on  T_priority=High  T=T_init_window degC  T_nominal_specify=off  T_nominal_unit=K  T_nominal_value=1  Q_specify=off  Q_priority=None  Q=0 W  Q_nominal_specify=off  Q_nominal_unit=W  Q_nominal_value=1
      settings: SourceProductBaseCode=PW,SS,VE
  Window-Exterior Conduction : fl_lib/Thermal/Thermal Elements/Conductive Heat Transfer  area=area_window m^2  thickness=thickness_window / 2 m  th_cond=k_window W/(K*m)  T_specify=off  T_priority=None  T=0 K  T_nominal_specify=off  T_nominal_unit=K  T_nominal_value=1  Q_specify=off  Q_priority=None  Q=0 W  Q_nominal_specify=off  Q_nominal_unit=W  Q_nominal_value=1
      settings: SourceProductBaseCode=PW,SS,VE
  Window-Exterior Convection : fl_lib/Thermal/Thermal Elements/Convective Heat Transfer  area=area_window m^2  heat_tr_coeff=hc_window_exterior W/(K*m^2)  T_specify=off  T_priority=None  T=0 K  T_nominal_specify=off  T_nominal_unit=K  T_nominal_value=1  Q_specify=off  Q_priority=None  Q=0 W  Q_nominal_specify=off  Q_nominal_unit=W  Q_nominal_value=1
      settings: SourceProductBaseCode=PW,SS,VE
  Window-Interior Conduction : fl_lib/Thermal/Thermal Elements/Conductive Heat Transfer  area=area_window m^2  thickness=thickness_window / 2 m  th_cond=k_window W/(K*m)  T_specify=off  T_priority=None  T=0 K  T_nominal_specify=off  T_nominal_unit=K  T_nominal_value=1  Q_specify=off  Q_priority=None  Q=0 W  Q_nominal_specify=off  Q_nominal_unit=W  Q_nominal_value=1
      settings: SourceProductBaseCode=PW,SS,VE
  Window-Interior Convection : fl_lib/Thermal/Thermal Elements/Convective Heat Transfer  area=area_window m^2  heat_tr_coeff=hc_window_interior W/(K*m^2)  T_specify=off  T_priority=None  T=0 K  T_nominal_specify=off  T_nominal_unit=K  T_nominal_value=1  Q_specify=off  Q_priority=None  Q=0 W  Q_nominal_specify=off  Q_nominal_unit=W  Q_nominal_value=1
      settings: SourceProductBaseCode=PW,SS,VE
  Exterior : PMIOPort  Side=Left
  Interior : PMIOPort  Port=2  Side=Right
  connections:
  Roof-Interior Convection/LConn1 -- Roof-Interior Conduction/RConn1
  Roof-Exterior Conduction/RConn1 -- Roof-Interior Conduction/LConn1 -- Roof Thermal Mass/LConn1
  Wall Thermal Mass SE/LConn1 -- Wall-Exterior Conduction SE/RConn1 -- Wall-Interior Conduction SE/LConn1
  Wall-Interior Conduction SE/RConn1 -- Wall-Interior Convection SE/LConn1
  Window-Interior Conduction/RConn1 -- Window-Interior Convection/LConn1
  Window-Exterior Conduction/RConn1 -- Window-Interior Conduction/LConn1 -- Window Thermal Mass/LConn1
  Wall-Exterior Conduction SE/LConn1 -- Wall-Exterior Convection SE/RConn1
  Furniture-Interior Convection/RConn1 -- Wall-Interior Convection SW/RConn1 -- Wall-Interior Convection  NW/RConn1 -- Wall-Interior Convection SE/RConn1 -- Roof-Interior Convection/RConn1 -- Wall-Interior Convection NE/RConn1 -- Interior/RConn1 -- Window-Interior Convection/RConn1
  Roof-Exterior Convection/LConn1 -- Wall-Exterior Convection SE/LConn1 -- Wall-Exterior Convection NE/LConn1 -- Wall-Exterior Convection NW/LConn1 -- Wall-Exterior Convection SW/LConn1 -- Exterior/RConn1 -- Window-Exterior Convection/LConn1
  Furniture-Interior Convection/LConn1 -- Furniture Thermal Mass/LConn1
  Roof-Exterior Conduction/LConn1 -- Roof-Exterior Convection/RConn1
  Window-Exterior Conduction/LConn1 -- Window-Exterior Convection/RConn1
  Wall Thermal Mass NE/LConn1 -- Wall-Exterior Conduction NE/RConn1 -- Wall-Interior Conduction NE/LConn1
  Wall-Exterior Conduction NE/LConn1 -- Wall-Exterior Convection NE/RConn1
  Wall-Interior Conduction NE/RConn1 -- Wall-Interior Convection NE/LConn1
  Wall-Exterior Conduction  NW/RConn1 -- Wall Thermal Mass  NW/LConn1 -- Wall-Interior Conduction  NW/LConn1
  Wall-Interior Conduction  NW/RConn1 -- Wall-Interior Convection  NW/LConn1
  Wall-Exterior Conduction  NW/LConn1 -- Wall-Exterior Convection NW/RConn1
  Wall Thermal Mass SW/LConn1 -- Wall-Exterior Conduction SW/RConn1 -- Wall-Interior Conduction SW/LConn1
  Wall-Interior Conduction SW/RConn1 -- Wall-Interior Convection SW/LConn1
  Wall-Exterior Conduction SW/LConn1 -- Wall-Exterior Convection SW/RConn1

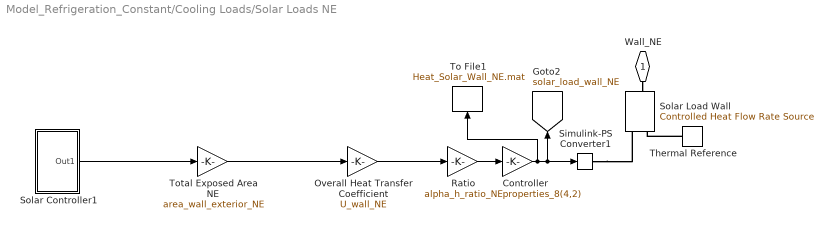
== system Model_Refrigeration_Constant/Cooling Loads/Solar Loads NE ==
  Controller : Gain  Gain=properties_8(4,2)
  Overall Heat Transfer Coefficient : Gain  Gain=U_wall_NE
  "Ratio " : Gain  Gain=alpha_h_ratio_NE
  Simulink-PS Converter1 : nesl_utility/Simulink-PS Converter  PhysicalDomain=network_engine_domain  SubClassName=ps_input  LeftPortType=input  RightPortType=output  PseudoPeriodic=off  Frequencies=[]  NoiseDistribution=none  NoiseParameters=[]  Unit=1  AffineConversion=off  FilteringAndDerivatives=provide  SimscapeFilterOrder=1  InputFilterTimeConstant=0.001  UdotUserProvided=0
      settings: SourceProductBaseCode=SS,PW,VE
  Solar Controller1 : Subsystem
  Solar Load Wall : fl_lib/Thermal/Thermal Sources/Controlled Heat Flow Rate Source
      settings: SourceProductBaseCode=PW,SS,VE
  Thermal Reference : fl_lib/Thermal/Thermal Elements/Thermal Reference
      settings: SourceProductBaseCode=PW,SS,VE
  To File1 : ToFile  Filename=Heat_Solar_Wall_NE.mat  MatrixName=Heat_Solar_Wall_NE
  Total Exposed Area NE : Gain  Gain=area_wall_exterior_NE
  Wall_NE : PMIOPort  Side=Right
  tag scope: solar_load_wall_NE=global
  wires:
  Total Exposed Area NE/1 -> Overall Heat Transfer Coefficient/1
  Overall Heat Transfer Coefficient/1 -> "Ratio "/1
  "Ratio "/1 -> Controller/1
  Controller/1 -> To File1/1, [solar_load_wall_NE], Simulink-PS Converter1/1
  Solar Controller1/1(Out1) -> Total Exposed Area NE/1
  connections:
  Simulink-PS Converter1/RConn1 -- Solar Load Wall/RConn1
  Thermal Reference/LConn1 -- Solar Load Wall/RConn2
  Wall_NE/RConn1 -- Solar Load Wall/LConn1

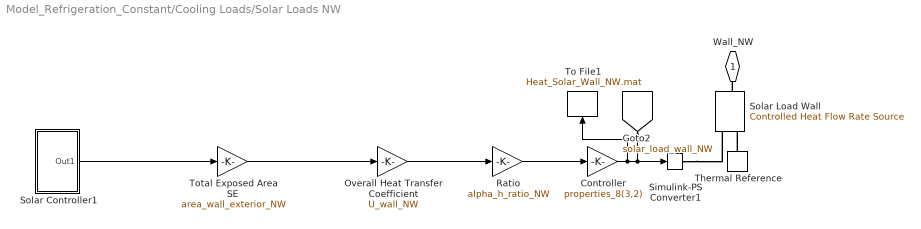
== system Model_Refrigeration_Constant/Cooling Loads/Solar Loads NW ==
  Controller : Gain  Gain=properties_8(3,2)
  Overall Heat Transfer Coefficient : Gain  Gain=U_wall_NW
  "Ratio " : Gain  Gain=alpha_h_ratio_NW
  Simulink-PS Converter1 : nesl_utility/Simulink-PS Converter  PhysicalDomain=network_engine_domain  SubClassName=ps_input  LeftPortType=input  RightPortType=output  PseudoPeriodic=off  Frequencies=[]  NoiseDistribution=none  NoiseParameters=[]  Unit=1  AffineConversion=off  FilteringAndDerivatives=provide  SimscapeFilterOrder=1  InputFilterTimeConstant=0.001  UdotUserProvided=0
      settings: SourceProductBaseCode=SS,PW,VE
  Solar Controller1 : Subsystem
  Solar Load Wall : fl_lib/Thermal/Thermal Sources/Controlled Heat Flow Rate Source
      settings: SourceProductBaseCode=PW,SS,VE
  Thermal Reference : fl_lib/Thermal/Thermal Elements/Thermal Reference
      settings: SourceProductBaseCode=PW,SS,VE
  To File1 : ToFile  Filename=Heat_Solar_Wall_NW.mat  MatrixName=Heat_Solar_Wall_NW
  Total Exposed Area SE : Gain  Gain=area_wall_exterior_NW
  Wall_NW : PMIOPort  Side=Right
  tag scope: solar_load_wall_NW=global
  wires:
  Total Exposed Area SE/1 -> Overall Heat Transfer Coefficient/1
  Overall Heat Transfer Coefficient/1 -> "Ratio "/1
  "Ratio "/1 -> Controller/1
  Controller/1 -> To File1/1, [solar_load_wall_NW], Simulink-PS Converter1/1
  Solar Controller1/1(Out1) -> Total Exposed Area SE/1
  connections:
  Simulink-PS Converter1/RConn1 -- Solar Load Wall/RConn1
  Solar Load Wall/LConn1 -- Wall_NW/RConn1
  Thermal Reference/LConn1 -- Solar Load Wall/RConn2

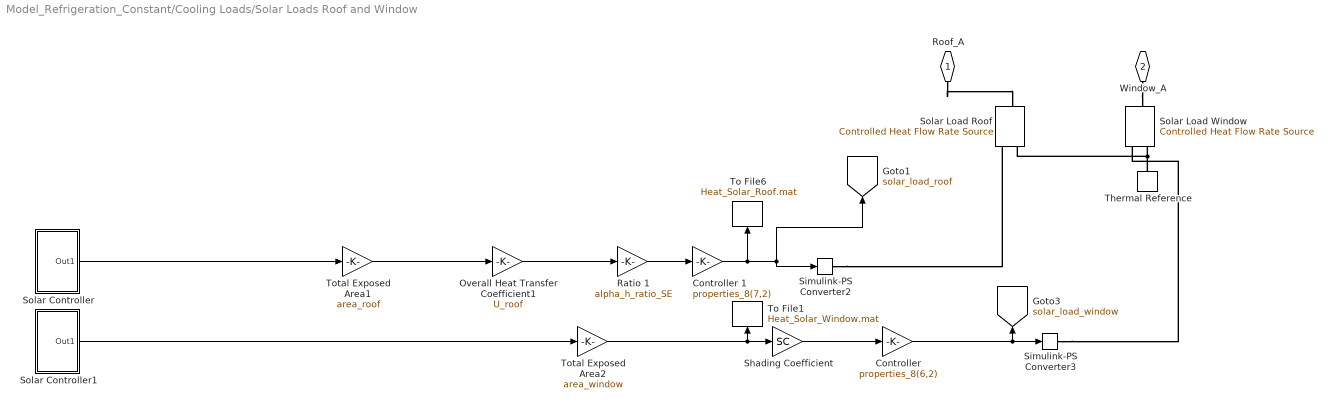
== system Model_Refrigeration_Constant/Cooling Loads/Solar Loads Roof and Window ==
  Controller : Gain  Gain=properties_8(6,2)
  Controller 1 : Gain  Gain=properties_8(7,2)
  Overall Heat Transfer Coefficient1 : Gain  Gain=U_roof
  Ratio 1 : Gain  Gain=alpha_h_ratio_SE
  Shading Coefficient : Gain  Gain=SC
  Simulink-PS Converter2 : nesl_utility/Simulink-PS Converter  PhysicalDomain=network_engine_domain  SubClassName=ps_input  LeftPortType=input  RightPortType=output  PseudoPeriodic=off  Frequencies=[]  NoiseDistribution=none  NoiseParameters=[]  Unit=1  AffineConversion=off  FilteringAndDerivatives=provide  SimscapeFilterOrder=1  InputFilterTimeConstant=0.001  UdotUserProvided=0
      settings: SourceProductBaseCode=SS,PW,VE
  Simulink-PS Converter3 : nesl_utility/Simulink-PS Converter  PhysicalDomain=network_engine_domain  SubClassName=ps_input  LeftPortType=input  RightPortType=output  PseudoPeriodic=off  Frequencies=[]  NoiseDistribution=none  NoiseParameters=[]  Unit=1  AffineConversion=off  FilteringAndDerivatives=provide  SimscapeFilterOrder=1  InputFilterTimeConstant=0.001  UdotUserProvided=0
      settings: SourceProductBaseCode=SS,PW,VE
  Solar Controller : Subsystem
  Solar Controller1 : Subsystem
  Solar Load Roof : fl_lib/Thermal/Thermal Sources/Controlled Heat Flow Rate Source
      settings: SourceProductBaseCode=PW,SS,VE
  Solar Load Window : fl_lib/Thermal/Thermal Sources/Controlled Heat Flow Rate Source
      settings: SourceProductBaseCode=PW,SS,VE
  Thermal Reference : fl_lib/Thermal/Thermal Elements/Thermal Reference
      settings: SourceProductBaseCode=PW,SS,VE
  To File1 : ToFile  Filename=Heat_Solar_Window.mat  MatrixName=Heat_Solar_Window
  To File6 : ToFile  Filename=Heat_Solar_Roof.mat  MatrixName=Heat_Solar_Roof
  Total Exposed Area1 : Gain  Gain=area_roof
  Total Exposed Area2 : Gain  Gain=area_window
  Roof_A : PMIOPort  Side=Right
  Window_A : PMIOPort  Port=2  Side=Right
  tag scope: solar_load_roof=global, solar_load_window=global
  wires:
  Total Exposed Area2/1 -> To File1/1, Shading Coefficient/1
  Total Exposed Area1/1 -> Overall Heat Transfer Coefficient1/1
  Shading Coefficient/1 -> Controller/1
  Ratio 1/1 -> Controller 1/1
  Overall Heat Transfer Coefficient1/1 -> Ratio 1/1
  Controller/1 -> Simulink-PS Converter3/1, [solar_load_window]
  Controller 1/1 -> To File6/1, Simulink-PS Converter2/1, [solar_load_roof]
  Solar Controller/1(Out1) -> Total Exposed Area1/1
  Solar Controller1/1(Out1) -> Total Exposed Area2/1
  connections:
  Simulink-PS Converter2/RConn1 -- Solar Load Roof/RConn1
  Simulink-PS Converter3/RConn1 -- Solar Load Window/RConn1
  Roof_A/RConn1 -- Solar Load Roof/LConn1
  Window_A/RConn1 -- Solar Load Window/LConn1
  Thermal Reference/LConn1 -- Solar Load Roof/RConn2 -- Solar Load Window/RConn2

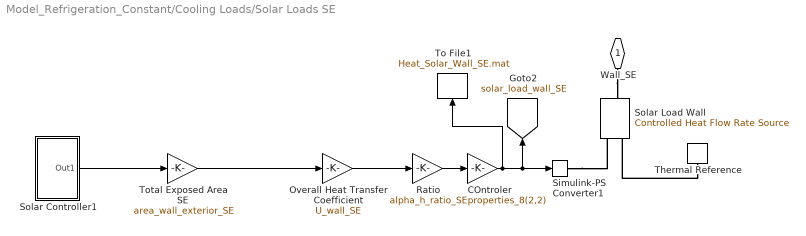
== system Model_Refrigeration_Constant/Cooling Loads/Solar Loads SE ==
  COntroler : Gain  Gain=properties_8(2,2)
  Overall Heat Transfer Coefficient : Gain  Gain=U_wall_SE
  "Ratio " : Gain  Gain=alpha_h_ratio_SE
  Simulink-PS Converter1 : nesl_utility/Simulink-PS Converter  PhysicalDomain=network_engine_domain  SubClassName=ps_input  LeftPortType=input  RightPortType=output  PseudoPeriodic=off  Frequencies=[]  NoiseDistribution=none  NoiseParameters=[]  Unit=1  AffineConversion=off  FilteringAndDerivatives=provide  SimscapeFilterOrder=1  InputFilterTimeConstant=0.001  UdotUserProvided=0
      settings: SourceProductBaseCode=SS,PW,VE
  Solar Controller1 : Subsystem
  Solar Load Wall : fl_lib/Thermal/Thermal Sources/Controlled Heat Flow Rate Source
      settings: SourceProductBaseCode=PW,SS,VE
  Thermal Reference : fl_lib/Thermal/Thermal Elements/Thermal Reference
      settings: SourceProductBaseCode=PW,SS,VE
  To File1 : ToFile  Filename=Heat_Solar_Wall_SE.mat  MatrixName=Heat_Solar_Wall_SE
  Total Exposed Area SE : Gain  Gain=area_wall_exterior_SE
  Wall_SE : PMIOPort  Side=Right
  tag scope: solar_load_wall_SE=global
  wires:
  Total Exposed Area SE/1 -> Overall Heat Transfer Coefficient/1
  Overall Heat Transfer Coefficient/1 -> "Ratio "/1
  "Ratio "/1 -> COntroler/1
  Solar Controller1/1(Out1) -> Total Exposed Area SE/1
  COntroler/1 -> To File1/1, [solar_load_wall_SE], Simulink-PS Converter1/1
  connections:
  Simulink-PS Converter1/RConn1 -- Solar Load Wall/RConn1
  Thermal Reference/LConn1 -- Solar Load Wall/RConn2
  Wall_SE/RConn1 -- Solar Load Wall/LConn1

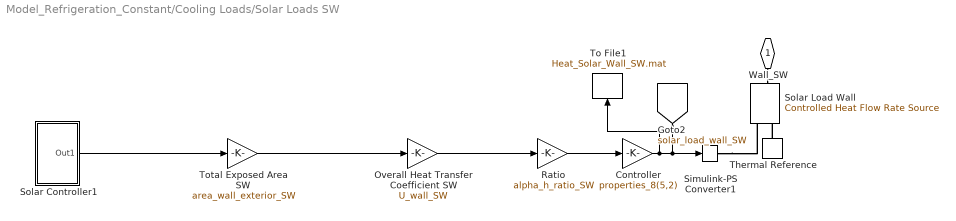
== system Model_Refrigeration_Constant/Cooling Loads/Solar Loads SW ==
  Controller : Gain  Gain=properties_8(5,2)
  Overall Heat Transfer Coefficient SW : Gain  Gain=U_wall_SW
  "Ratio " : Gain  Gain=alpha_h_ratio_SW
  Simulink-PS Converter1 : nesl_utility/Simulink-PS Converter  PhysicalDomain=network_engine_domain  SubClassName=ps_input  LeftPortType=input  RightPortType=output  PseudoPeriodic=off  Frequencies=[]  NoiseDistribution=none  NoiseParameters=[]  Unit=1  AffineConversion=off  FilteringAndDerivatives=provide  SimscapeFilterOrder=1  InputFilterTimeConstant=0.001  UdotUserProvided=0
      settings: SourceProductBaseCode=SS,PW,VE
  Solar Controller1 : Subsystem
  Solar Load Wall : fl_lib/Thermal/Thermal Sources/Controlled Heat Flow Rate Source
      settings: SourceProductBaseCode=PW,SS,VE
  Thermal Reference : fl_lib/Thermal/Thermal Elements/Thermal Reference
      settings: SourceProductBaseCode=PW,SS,VE
  To File1 : ToFile  Filename=Heat_Solar_Wall_SW.mat  MatrixName=Heat_Solar_Wall_SW
  Total Exposed Area SW : Gain  Gain=area_wall_exterior_SW
  Wall_SW : PMIOPort  Side=Right
  tag scope: solar_load_wall_SW=global
  wires:
  Total Exposed Area SW/1 -> Overall Heat Transfer Coefficient SW/1
  Overall Heat Transfer Coefficient SW/1 -> "Ratio "/1
  "Ratio "/1 -> Controller/1
  Controller/1 -> To File1/1, [solar_load_wall_SW], Simulink-PS Converter1/1
  Solar Controller1/1(Out1) -> Total Exposed Area SW/1
  connections:
  Simulink-PS Converter1/RConn1 -- Solar Load Wall/RConn1
  Thermal Reference/LConn1 -- Solar Load Wall/RConn2
  Wall_SW/RConn1 -- Solar Load Wall/LConn1

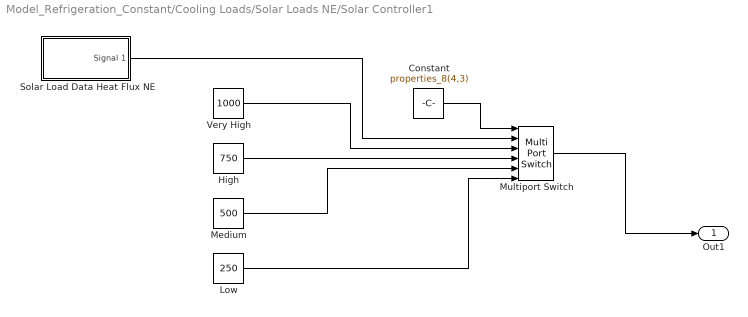
== system Model_Refrigeration_Constant/Cooling Loads/Solar Loads NE/Solar Controller1 ==
  Constant : Constant  Value=properties_8(4,3)
  "High " : Constant  Value=750
  Low : Constant  Value=250
  Medium : Constant  Value=500
  Multiport Switch : MultiPortSwitch  Inputs=5  SaturateOnIntegerOverflow=off  InputSameDT=off
  Solar Load Data Heat Flux NE : Subsystem  Tag=STV Subsys  LoadFcn=sigbuilder_block('load');  StartFcn=sigbuilder_block('start');  StopFcn=sigbuilder_block('stop');  ClipboardFcn=sigbuilder_block('clipboard');  mask(Sigbuilder block){tuvar=[0:10]}
      mask help: Simulink:masks:SigbuilderBlock_MD
      mask init:
      | if ~strcmp(get_param(bdroot(gcbh),'SimulationStatus'),'stopped') tuvar = sigbuilder_block('maskInit'); end
      settings: CopyFcn=sigbuilder_block('copy');  DeleteFcn=sigbuilder_block('delete');  ModelCloseFcn=sigbuilder_block('modelClose');  PreSaveFcn=sigbuilder_block('preSave');  PauseFcn=sigbuilder_block('pause');  ContinueFcn=sigbuilder_block('continue');  NameChangeFcn=sigbuilder_block('namechange');  OpenFcn=sigbuilder_block('open',[751.2 -47.4 395.4 359.4 ]);  CloseFcn=sigbuilder_block('close');
      mask Display: plot(0, 0, 100, 100,[2, 2, 32, 32, 2], [68, 8, 8, 68, 68],[32, 2], [38, 38], [32, 19, 2],[53, 60, 44], [32, 17, 17, 2],[16, 16, 31, 31]);txt = getActiveGroup(gcbh);text(2, 100, txt,'verticalAlignment', 'top');
  Very High : Constant  Value=1000
  Out1 : Outport
  wires:
  Very High/1 -> Multiport Switch/3
  Solar Load Data Heat Flux NE/1(Signal 1) -> Multiport Switch/2
  Multiport Switch/1 -> Out1/1
  Constant/1 -> Multiport Switch/1
  "High "/1 -> Multiport Switch/4
  Medium/1 -> Multiport Switch/5
  Low/1 -> Multiport Switch/6

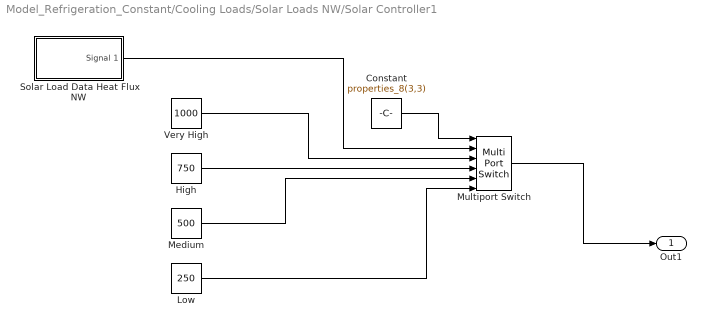
== system Model_Refrigeration_Constant/Cooling Loads/Solar Loads NW/Solar Controller1 ==
  Constant : Constant  Value=properties_8(3,3)
  "High " : Constant  Value=750
  Low : Constant  Value=250
  Medium : Constant  Value=500
  Multiport Switch : MultiPortSwitch  Inputs=5  SaturateOnIntegerOverflow=off  InputSameDT=off
  Solar Load Data Heat Flux NW : Subsystem  Tag=STV Subsys  LoadFcn=sigbuilder_block('load');  StartFcn=sigbuilder_block('start');  StopFcn=sigbuilder_block('stop');  ClipboardFcn=sigbuilder_block('clipboard');  mask(Sigbuilder block){tuvar=[0:10]}
      mask help: Simulink:masks:SigbuilderBlock_MD
      mask init:
      | if ~strcmp(get_param(bdroot(gcbh),'SimulationStatus'),'stopped') tuvar = sigbuilder_block('maskInit'); end
      settings: CopyFcn=sigbuilder_block('copy');  DeleteFcn=sigbuilder_block('delete');  ModelCloseFcn=sigbuilder_block('modelClose');  PreSaveFcn=sigbuilder_block('preSave');  PauseFcn=sigbuilder_block('pause');  ContinueFcn=sigbuilder_block('continue');  NameChangeFcn=sigbuilder_block('namechange');  OpenFcn=sigbuilder_block('open',[470.4 201 394.8 282 ]);  CloseFcn=sigbuilder_block('close');
      mask Display: plot(0, 0, 100, 100,[2, 2, 32, 32, 2], [68, 8, 8, 68, 68],[32, 2], [38, 38], [32, 19, 2],[53, 60, 44], [32, 17, 17, 2],[16, 16, 31, 31]);txt = getActiveGroup(gcbh);text(2, 100, txt,'verticalAlignment', 'top');
  Very High : Constant  Value=1000
  Out1 : Outport
  wires:
  Very High/1 -> Multiport Switch/3
  Multiport Switch/1 -> Out1/1
  Constant/1 -> Multiport Switch/1
  "High "/1 -> Multiport Switch/4
  Medium/1 -> Multiport Switch/5
  Low/1 -> Multiport Switch/6
  Solar Load Data Heat Flux NW/1(Signal 1) -> Multiport Switch/2

== system Model_Refrigeration_Constant/Cooling Loads/Solar Loads Roof and Window/Solar Controller ==
  Constant : Constant  Value=properties_8(7,3)
  "High " : Constant  Value=750
  Low : Constant  Value=250
  Medium : Constant  Value=500
  Multiport Switch : MultiPortSwitch  Inputs=5  SaturateOnIntegerOverflow=off  InputSameDT=off
  Solar Load Data Heat Roof : Subsystem  Tag=STV Subsys  LoadFcn=sigbuilder_block('load');  StartFcn=sigbuilder_block('start');  StopFcn=sigbuilder_block('stop');  ClipboardFcn=sigbuilder_block('clipboard');  mask(Sigbuilder block){tuvar=[0:10]}
      mask help: Simulink:masks:SigbuilderBlock_MD
      mask init:
      | if ~strcmp(get_param(bdroot(gcbh),'SimulationStatus'),'stopped') tuvar = sigbuilder_block('maskInit'); end
      settings: CopyFcn=sigbuilder_block('copy');  DeleteFcn=sigbuilder_block('delete');  ModelCloseFcn=sigbuilder_block('modelClose');  PreSaveFcn=sigbuilder_block('preSave');  PauseFcn=sigbuilder_block('pause');  ContinueFcn=sigbuilder_block('continue');  NameChangeFcn=sigbuilder_block('namechange');  OpenFcn=sigbuilder_block('open',[376.8 216 395.4 359.4 ]);  CloseFcn=sigbuilder_block('close');
      mask Display: plot(0, 0, 100, 100,[2, 2, 32, 32, 2], [68, 8, 8, 68, 68],[32, 2], [38, 38], [32, 19, 2],[53, 60, 44], [32, 17, 17, 2],[16, 16, 31, 31]);txt = getActiveGroup(gcbh);text(2, 100, txt,'verticalAlignment', 'top');
  Very High : Constant  Value=1000
  Out1 : Outport
  wires:
  Low/1 -> Multiport Switch/6
  Medium/1 -> Multiport Switch/5
  "High "/1 -> Multiport Switch/4
  Constant/1 -> Multiport Switch/1
  Multiport Switch/1 -> Out1/1
  Solar Load Data Heat Roof/1(Signal 1) -> Multiport Switch/2
  Very High/1 -> Multiport Switch/3
